simulink library "Surface_Profile_Axle3_zx_LR"  (R2025a)
settings: Solver=VariableStepAuto  StartTime=0.0  StopTime=10.0  RelTol=1e-3
Description:
  | Simscape Vehicle Templates Library
  | 
  | Copyright 2018-2025 The MathWorks, Inc.
settings Model: Creator=smiller  LastModifiedBy=smiller
settings ModelReferenceCC: EnableRefExpFcnMdlSchedulingChecks=on
settings RTWCC: GPUComputeCapability=3.5

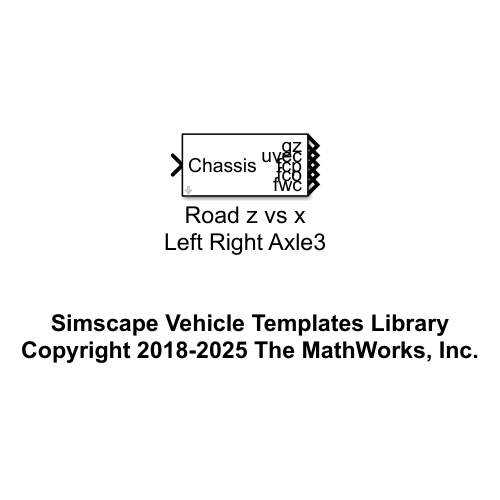
[thumbnail: Simulink's stored preview of the top-level diagram]
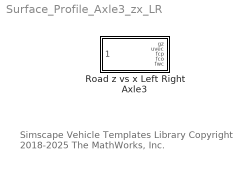
== system Surface_Profile_Axle3_zx_LR ==
  note: Simscape Vehicle Templates Library
      | Copyright 2018-2025 The MathWorks, Inc.
  Road z vs x Left Right Axle3 : Subsystem  VariantControl=Variant  mask{dist_x_l=flipud(Scene.RDF_Plateau.Road.extr_data_L(45:end,1)), height_z_l=flipud(Scene.RDF_Plateau.Road.extr_data_L(45:end,2)), dist_x_r=flipud(Scene.RDF_Plateau.Road.extr_data_R(45:end,1)), height_z_r=flipud(Scene.RDF_Plateau.Road.extr_data_R(45:end,2))}
      mask prompts: dist_x_l "Distance Vector Left [x] (m)"; height_z_l "Height Vector Left [z] (m)"; dist_x_r "Distance Vector Right [x] (m)"; height_z_r "Height Vector Right [z] (m)"
      mask init:
      | pitch_l = atan2(circshift(height_z_l,-2)-circshift(height_z_l,2),circshift(dist_x_l,-2)-circshift(dist_x_l,2));
      | pitch_l(1:2) = pitch_l(3);
      | pitch_l(end-1:end) = pitch_l(end-2);
      | 
      | pitch_r = atan2(circshift(height_z_r,-2)-circshift(height_z_r,2),circshift(dist_x_r,-2)-circshift(dist_x_r,2));
      | pitch_r(1:2) = pitch_r(3);
      | pitch_r(end-1:end) = pitch_r(end-2);

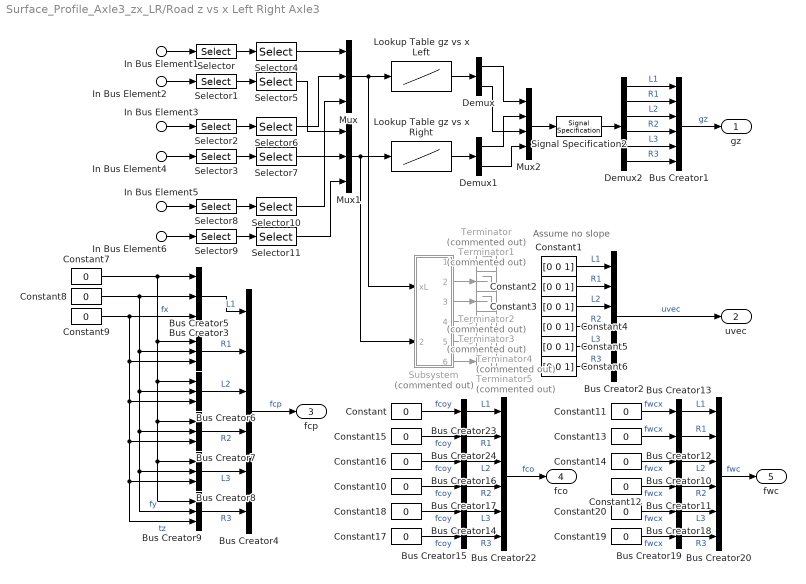
== system Surface_Profile_Axle3_zx_LR/Road z vs x Left Right Axle3 ==
  note: Assume no slope
  In Bus Element1 : Inport  PortName=Chassis  Element=WhlL1.xyz
  In Bus Element2 : Inport  PortName=Chassis  Element=WhlR1.xyz
  In Bus Element3 : Inport  PortName=Chassis  Element=WhlL2.xyz
  In Bus Element4 : Inport  PortName=Chassis  Element=WhlR2.xyz
  In Bus Element5 : Inport  PortName=Chassis  Element=WhlL3.xyz
  In Bus Element6 : Inport  PortName=Chassis  Element=WhlR3.xyz
  Bus Creator{1..2,4,20,22} (5 alike) : BusCreator  Inputs=6
  Bus Creator{10..19,23..24} (12 alike) : BusCreator  Inputs=1
  Bus Creator{3,5..9} (6 alike) : BusCreator  Inputs=3
  Constant{,7..20} (15 alike) : Constant  Value=0
  Constant{1..6} (6 alike) : Constant  Value=[0 0 1]
  Demux : Demux  Outputs=2
  Demux1 : Demux  Outputs=2
  Demux2 : Demux  Outputs=6
  Lookup Table gz vs x Left : Lookup_n-D  NumberOfTableDimensions=1  BreakpointsForDimension1=dist_x_l  Table=height_z_l  InternalRulePriority=Speed  RndMeth=Simplest
  Lookup Table gz vs x Right : Lookup_n-D  NumberOfTableDimensions=1  BreakpointsForDimension1=dist_x_r  Table=height_z_r  InternalRulePriority=Speed  RndMeth=Simplest
  Mux : Mux  Inputs=3
  Mux1 : Mux  Inputs=3
  Mux2 : Mux
  Selector{,1..3,8..9} (6 alike) : Selector  InputPortWidth=3  IndexOptions=Index vector (dialog)  Indices=[1 2]  OutputSizes=1
  Selector{4..7,10..11} (6 alike) : Selector  InputPortWidth=2  IndexOptions=Index vector (dialog)  Indices=1  OutputSizes=1
  Signal Specification2 : SignalSpecification  Unit=m
  Subsystem : Subsystem  Commented=on
  Terminator{,1..5} (6 alike) : Terminator  Commented=on
  gz : Outport  VectorParamsAs1DForOutWhenUnconnected=off
  uvec : Outport  Port=2  VectorParamsAs1DForOutWhenUnconnected=off
  fcp : Outport  Port=3  VectorParamsAs1DForOutWhenUnconnected=off
  fco : Outport  Port=4  VectorParamsAs1DForOutWhenUnconnected=off
  fwc : Outport  Port=5  VectorParamsAs1DForOutWhenUnconnected=off
  wires:
  Subsystem/6(R3) -> Terminator5/1
  Subsystem/5(L3) -> Terminator4/1
  Constant6/1 -> Bus Creator2/6  "R3"
  Constant5/1 -> Bus Creator2/5  "L3"
  Demux2/6 -> Bus Creator1/6  "R3"
  Demux2/5 -> Bus Creator1/5  "L3"
  Selector11/1 -> Mux1/3
  Selector10/1 -> Mux/3
  Selector9/1 -> Selector11/1
  Selector8/1 -> Selector10/1
  In Bus Element6/1 -> Selector9/1
  In Bus Element5/1 -> Selector8/1
  Signal Specification2/1 -> Demux2/1
  In Bus Element3/1 -> Selector2/1
  In Bus Element1/1 -> Selector/1
  In Bus Element2/1 -> Selector1/1
  In Bus Element4/1 -> Selector3/1
  Selector/1 -> Selector4/1
  Selector1/1 -> Selector5/1
  Selector2/1 -> Selector6/1
  Selector3/1 -> Selector7/1
  Selector7/1 -> Mux1/2
  Selector6/1 -> Mux/2
  Selector5/1 -> Mux1/1
  Selector4/1 -> Mux/1
  Lookup Table gz vs x Right/1 -> Demux1/1
  Lookup Table gz vs x Left/1 -> Demux/1
  Demux/1 -> Mux2/1
  Demux1/1 -> Mux2/2
  Demux/2 -> Mux2/3
  Demux1/2 -> Mux2/4
  Mux2/1 -> Signal Specification2/1
  Mux1/1 -> Subsystem/2(xR), Lookup Table gz vs x Right/1
  Mux/1 -> Subsystem/1(xL), Lookup Table gz vs x Left/1
  Demux2/1 -> Bus Creator1/1  "L1"
  Demux2/2 -> Bus Creator1/2  "R1"
  Demux2/3 -> Bus Creator1/3  "L2"
  Demux2/4 -> Bus Creator1/4  "R2"
  Bus Creator1/1 -> gz/1  "gz"
  Constant1/1 -> Bus Creator2/1  "L1"
  Constant3/1 -> Bus Creator2/3  "L2"
  Constant2/1 -> Bus Creator2/2  "R1"
  Bus Creator2/1 -> uvec/1  "uvec"
  Constant4/1 -> Bus Creator2/4  "R2"
  Subsystem/1(L1) -> Terminator/1
  Subsystem/4(R2) -> Terminator3/1
  Subsystem/2(R1) -> Terminator1/1
  Subsystem/3(L2) -> Terminator2/1
  Bus Creator8/1 -> Bus Creator4/5  "L3"
  Constant8/1 -> Bus Creator3/2, Bus Creator5/2, Bus Creator6/2, Bus Creator7/2, Bus Creator8/2, Bus Creator9/2  "fy"
  Constant7/1 -> Bus Creator3/1, Bus Creator5/1, Bus Creator6/1, Bus Creator9/1, Bus Creator8/1, Bus Creator7/1  "fx"
  Bus Creator9/1 -> Bus Creator4/6  "R3"
  Bus Creator5/1 -> Bus Creator4/2  "R1"
  Bus Creator3/1 -> Bus Creator4/1  "L1"
  Bus Creator7/1 -> Bus Creator4/4  "R2"
  Bus Creator6/1 -> Bus Creator4/3  "L2"
  Bus Creator4/1 -> fcp/1  "fcp"
  Constant9/1 -> Bus Creator3/3, Bus Creator5/3, Bus Creator6/3, Bus Creator7/3, Bus Creator8/3, Bus Creator9/3  "tz"
  Constant20/1 -> Bus Creator18/1  "fwcx"
  Constant13/1 -> Bus Creator12/1  "fwcx"
  Constant15/1 -> Bus Creator24/1  "fcoy"
  Bus Creator10/1 -> Bus Creator20/3  "L2"
  Constant10/1 -> Bus Creator17/1  "fcoy"
  Bus Creator13/1 -> Bus Creator20/1  "L1"
  Bus Creator23/1 -> Bus Creator22/1  "L1"
  Bus Creator17/1 -> Bus Creator22/4  "R2"
  Constant14/1 -> Bus Creator10/1  "fwcx"
  Bus Creator22/1 -> fco/1  "fco"
  Constant17/1 -> Bus Creator15/1  "fcoy"
  Bus Creator15/1 -> Bus Creator22/6  "R3"
  Bus Creator14/1 -> Bus Creator22/5  "L3"
  Bus Creator18/1 -> Bus Creator20/5  "L3"
  Constant12/1 -> Bus Creator11/1  "fwcx"
  Bus Creator20/1 -> fwc/1  "fwc"
  Constant18/1 -> Bus Creator14/1  "fcoy"
  Bus Creator19/1 -> Bus Creator20/6  "R3"
  Bus Creator24/1 -> Bus Creator22/2  "R1"
  Constant16/1 -> Bus Creator16/1  "fcoy"
  Bus Creator16/1 -> Bus Creator22/3  "L2"
  Constant19/1 -> Bus Creator19/1  "fwcx"
  Constant11/1 -> Bus Creator13/1  "fwcx"
  Constant/1 -> Bus Creator23/1  "fcoy"
  Bus Creator12/1 -> Bus Creator20/2  "R1"
  Bus Creator11/1 -> Bus Creator20/4  "R2"

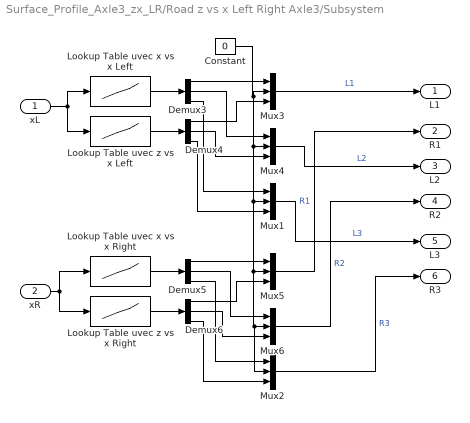
== system Surface_Profile_Axle3_zx_LR/Road z vs x Left Right Axle3/Subsystem ==
  xL : Inport
  xR : Inport  Port=2
  Constant : Constant  Value=0
  Demux{3..6} (4 alike) : Demux  Outputs=3
  Lookup Table uvec x vs x Left : Lookup_n-D  NumberOfTableDimensions=1  BreakpointsForDimension1=dist_x_l  Table=sin(pitch_l)  InternalRulePriority=Speed  RndMeth=Simplest
  Lookup Table uvec x vs x Right : Lookup_n-D  NumberOfTableDimensions=1  BreakpointsForDimension1=dist_x_r  Table=sin(pitch_r)  InternalRulePriority=Speed  RndMeth=Simplest
  Lookup Table uvec z vs x Left : Lookup_n-D  NumberOfTableDimensions=1  BreakpointsForDimension1=dist_x_l  Table=cos(pitch_l)  InternalRulePriority=Speed  RndMeth=Simplest
  Lookup Table uvec z vs x Right : Lookup_n-D  NumberOfTableDimensions=1  BreakpointsForDimension1=dist_x_r  Table=cos(pitch_r)  InternalRulePriority=Speed  RndMeth=Simplest
  Mux{1..6} (6 alike) : Mux  Inputs=3
  L1 : Outport  VectorParamsAs1DForOutWhenUnconnected=off
  R1 : Outport  Port=2  VectorParamsAs1DForOutWhenUnconnected=off
  L2 : Outport  Port=3  VectorParamsAs1DForOutWhenUnconnected=off
  R2 : Outport  Port=4  VectorParamsAs1DForOutWhenUnconnected=off
  L3 : Outport  Port=5  VectorParamsAs1DForOutWhenUnconnected=off
  R3 : Outport  Port=6  VectorParamsAs1DForOutWhenUnconnected=off
  wires:
  Demux6/3 -> Mux2/3
  Demux5/3 -> Mux2/1
  Mux2/1 -> R3/1  "R3"
  Demux4/3 -> Mux1/3
  Mux1/1 -> L3/1  "L3"
  Demux3/3 -> Mux1/1
  Lookup Table uvec x vs x Left/1 -> Demux3/1
  xL/1 -> Lookup Table uvec x vs x Left/1, Lookup Table uvec z vs x Left/1
  Mux6/1 -> R2/1  "R2"
  Demux4/1 -> Mux3/3
  Mux3/1 -> L1/1  "L1"
  Demux6/2 -> Mux6/3
  xR/1 -> Lookup Table uvec x vs x Right/1, Lookup Table uvec z vs x Right/1
  Lookup Table uvec z vs x Left/1 -> Demux4/1
  Demux3/2 -> Mux4/1
  Demux3/1 -> Mux3/1
  Lookup Table uvec z vs x Right/1 -> Demux6/1
  Demux4/2 -> Mux4/3
  Constant/1 -> Mux5/2, Mux6/2, Mux2/2, Mux1/2, Mux4/2, Mux3/2
  Mux5/1 -> R1/1  "R1"
  Demux5/2 -> Mux6/1
  Demux6/1 -> Mux5/3
  Demux5/1 -> Mux5/1
  Lookup Table uvec x vs x Right/1 -> Demux5/1
  Mux4/1 -> L2/1  "L2"
